simulink model "DC_Charging_Sequence_Block_testing"  (R2024b)
settings: Solver=FixedStepDiscrete  StartTime=0.0  StopTime=10.0  FixedStep=0.01  RelTol=1e-3
undefined symbols (not defined in the file or in its folder): CCM, raptor_get_safe_string, raptor_xcp_function
libraries: Raptor_lib x37
(part 1 of 2)
settings Model: RaptorUIDSize=4  Raptor_Target=CCM-58NN-112-2403  Raptor_Calloc=NonVolatile (EEPROM)  Raptor_ecuaddr=11  RaptorBuildNum=-1  Creator=noahm  LastModifiedBy=malul
settings OptimizationCC: DefaultParameterBehavior=Inlined  UseSpecifiedMinMax=on  InlineInvariantSignals=on  EnhancedBackFolding=on  PassReuseOutputArgsAs=Individual arguments  InitFltsAndDblsToZero=on  NoFixptDivByZeroProtection=on  EfficientFloat2IntCast=on  OptimizeBlockOrder=speed  DifferentSizesBufferReuse=on  OptimizationCustomize=off  EfficientTunableParamExpr=on
settings DebuggingCC: UnderspecifiedInitializationDetection=Classic  MergeDetectMultiDrivingBlocksExec=none  InheritedTsInSrcMsg=none  ParameterTunabilityLossMsg=error
settings HardwareCC: TargetIntDivRoundTo=Zero  TargetEndianess=BigEndian  ProdEqTarget=off
settings ModelReferenceCC: PropagateSignalLabelsOutOfModel=off
settings SFSimCC: MATLABDynamicMemAlloc=off
settings RTWCC: Description=Raptor (tm)  SystemTargetFile=raptor.tlc  MakeCommand=raptor_make_rtw  TemplateMakefile=raptor_tmf
settings CodeAppCC: ForceParamTrailComments=on  IgnoreCustomStorageClasses=off  MaxIdLength=100  OperatorAnnotations=on  SimulinkDataObjDesc=on  SFDataObjDesc=on  InsertBlockDesc=on
settings STFCustomTargetCC: TargetLangStandard=C99 (ISO)  MultiwordLength=256  GenerateSampleERTMain=on  CombineOutputUpdateFcns=on  CombineSignalStateStructs=on  ERTCustomFileBanners=on  SupportComplex=off  SupportContinuousTime=off  SupportNonInlinedSFcns=off  RemoveResetFunc=on  MATLABClassNameForMDSCustomization=Simulink.SoftwareTarget.ERTCustomization  SystemTargetFile=raptor.tlc
settings ERTTargetCC: TargetLangStandard=C99 (ISO)  GenerateSampleERTMain=on  ParMdlRefBuildCompliant=off  CompOptLevelCompliant=off  ConcurrentExecutionCompliant=off  CombineSignalStateStructs=on  SupportComplex=off  ModelStepFunctionPrototypeControlCompliant=off  CPPClassGenCompliant=off  UseToolchainInfoCompliant=off  ERTCustomFileTemplate=example_file_process.tlc

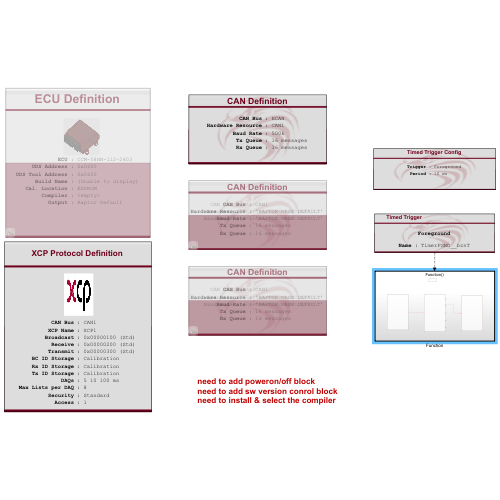
[thumbnail: Simulink's stored preview of the top-level diagram]
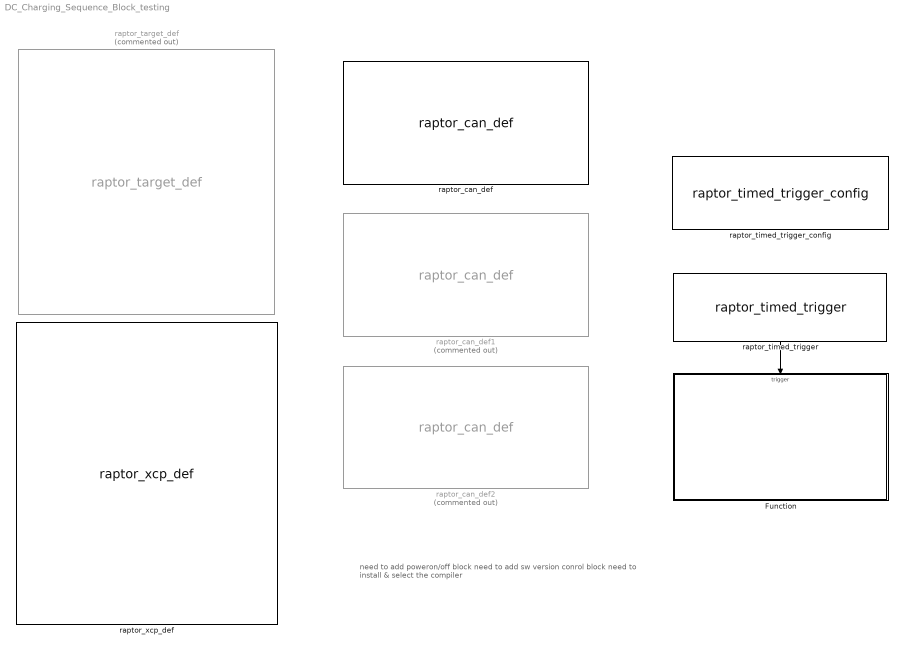
== system DC_Charging_Sequence_Block_testing ==
  note: need to add poweron/off block
      | need to add sw version conrol block
      | need to install & select the compiler
  Function : Subsystem
  raptor_can_def : Raptor_lib/CAN/raptor_can_def  canBus='HCAN'  resourceValues=CAN1|CAN2|CAN3|CAN4|CAN5|CAN6|CAN7|CAN8|(None)  resource=CAN1  baudRateValues=33k|50k|100k|125k|200k|250k|333k|500k|667k|800k|1000k  baudRate=500k  useCustomBR=0  customBR='CustomBaudRate'  enable_baud_rate_config=0  sim_func_name='ConfigureCANBaudRate'  createButton=0  updateButton=0  txQueueSize=16  rxQueueSize=16
      settings: SourceProductName=Raptor
  raptor_can_def1 : Raptor_lib/CAN/raptor_can_def  Commented=on  canBus='CAN1'  resourceValues=CAN1|CAN2|CAN3|CAN4|CAN5|CAN6|CAN7|CAN8|(None)  resource='RAPTOR MASK DEFAULT'  baudRateValues=(None)  baudRate='RAPTOR MASK DEFAULT'  useCustomBR=0  customBR='CustomBaudRate'  enable_baud_rate_config=0  sim_func_name='ConfigureCANBaudRate'  createButton=[]  updateButton=[]  txQueueSize=16  rxQueueSize=16
      settings: SourceProductName=Raptor
  raptor_can_def2 : Raptor_lib/CAN/raptor_can_def  Commented=on  canBus='CAN1'  resourceValues=CAN1|CAN2|CAN3|CAN4|CAN5|CAN6|CAN7|CAN8|(None)  resource='RAPTOR MASK DEFAULT'  baudRateValues=(None)  baudRate='RAPTOR MASK DEFAULT'  useCustomBR=0  customBR='CustomBaudRate'  enable_baud_rate_config=0  sim_func_name='ConfigureCANBaudRate'  createButton=[]  updateButton=[]  txQueueSize=16  rxQueueSize=16
      settings: SourceProductName=Raptor
  raptor_target_def : Raptor_lib/Configuration/raptor_target_def  Commented=on  targetValues=CCM-58NN-112-2403|CCM-TC377-112-2403|DISP-VC128-1901|DISP-VC320L-1402|DISP-VC320-1204|DISP-VC800-1402|DISP-VC500-1904|DISP-VC700-2003|DISP-VC300R-2004|GCM-5634M-070-1559|GCM-5634M-070-1562|EOL-58NN-176-2204|ECM-1793-196-1503|GCM-1793-196-1503|GCM-5605B-048-1906|GCM-5605B-048-2104|RCM-5743R-080-2203|RCM-5743R-080-2304|UAS-5743R-047-2102|UAS-5743R-047-2107|RCM-58NN-112-2103|RCM-58NN-112-2202|RCM-58NN-112-2208|RCM-58NN-112-2410|GCM-TC234-044-2409|GCM-TC277-106-2407|GCM-TC277-108-2406|GCM-TC337-056-2402|GCM-TC367-111-2301|HCM-5604-036-1303|HCM-5604-036-1702  target=CCM-58NN-112-2403  simpack=0  simulator=0  heap=2*1024  stack=4*1024  fgndStack=2*1024  bgndStack=2*1024  idleStack=1024  intStack=1536  sdStack=1024  appStack=1024  ecuaddr=11  uds_server_addr_ext=0  uds_server_addr=hex2dec('600')  uds_client_addr=hex2dec('650')  callocValues=Constant (FLASH)|NonVolatile (EEPROM)  calloc=NonVolatile (EEPROM)  compilerValues=[]  compiler=<empty>  setFileName=0  exeName=[raptor_get_safe_string(bdroot) '_']  addBuildNum=0  minVerChars=3  extraOutput=1  buildLocationValues=Raptor Default|Model Directory|User Defined  buildLocation=Raptor Default  exeLocation=''  exeFileButton=0  a2lLocation=''  a2lFileButton=0  rpgLocation=''  rpgFileButton=0
      settings: SourceProductName=Raptor
  raptor_timed_trigger : Raptor_lib/Triggers/raptor_timed_trigger  triggerValues=[]  trigger=Foreground  inherited=0  alwaysEnabled=1  triggerPriority=0  triggerName=FGND__bznT
      settings: SourceProductName=Raptor
  raptor_timed_trigger_config : Raptor_lib/Triggers/raptor_timed_trigger_config  triggerValues=Foreground|Background  trigger=Foreground  period=10
      settings: SourceProductName=Raptor
  raptor_xcp_def : Raptor_lib/Configuration/raptor_xcp_def  XCPname='XCP1'  canBus='CAN1'  bcID=hex2dec('100')  bcID_TypeValues=[]  bcID_Type=Standard  rxID=hex2dec('200')  rxID_TypeValues=[]  rxID_Type=Standard  txID=hex2dec('300')  txID_TypeValues=[]  txID_Type=Standard  daqRates=[5 10 100]  numODTs=8  genCANAPE=0  genVISION=0  securityValues=[]  security=Standard  dllName=raptor_XCPSecurity.dll  accessValues=[]  access=1  bcStorageValues=[]  bcStorage=Calibration  txStorageValues=[]  txStorage=Calibration  rxStorageValues=[]  rxStorage=Calibration
      settings: SourceProductName=Raptor
  wires:
  raptor_timed_trigger/1 -> Function/Trigger

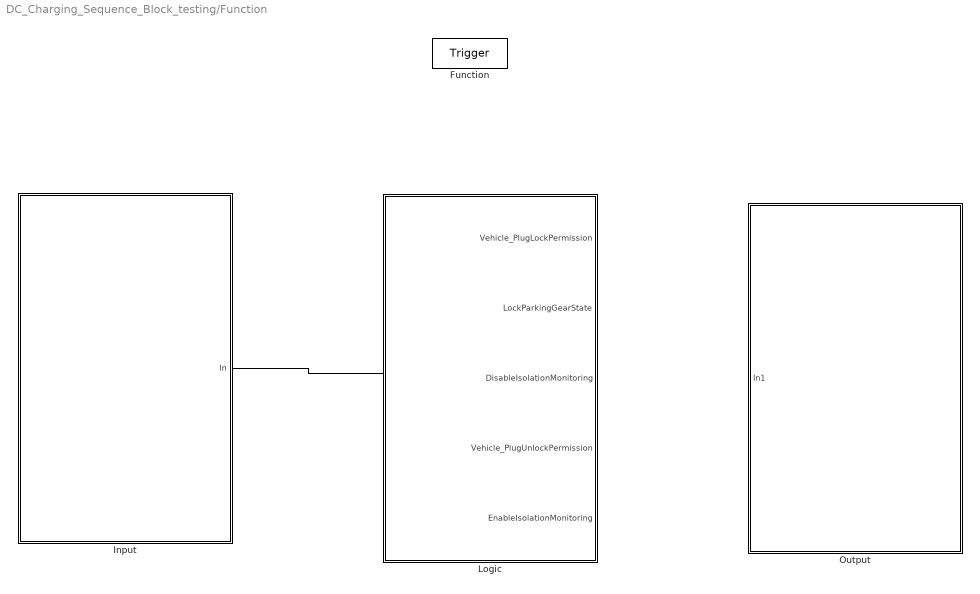
== system DC_Charging_Sequence_Block_testing/Function ==
  Function : TriggerPort  TriggerType=function-call  VariantControl=(inherit)  PortDimensions=1
  Input : Subsystem
  Logic : Subsystem
  Output : Subsystem
  wires:
  Input/1(In) -> ?
  ? -> Output/1(In1)

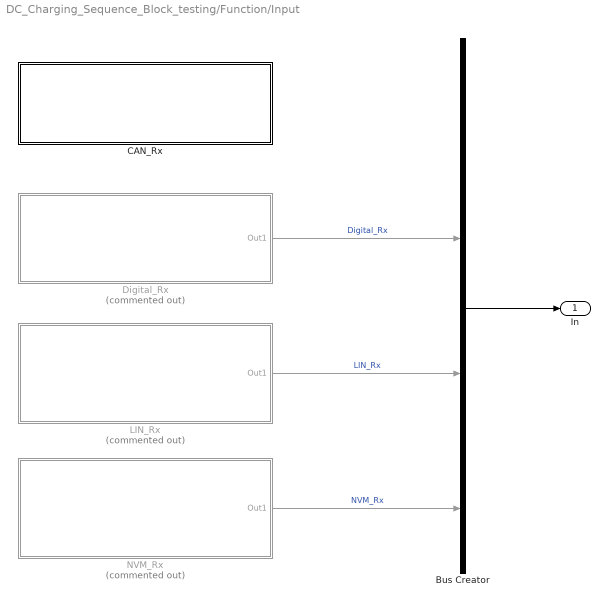
== system DC_Charging_Sequence_Block_testing/Function/Input ==
  Bus Creator : BusCreator  Inputs=4
  CAN_Rx : Subsystem
  Digital_Rx : Subsystem  Commented=on
  LIN_Rx : Subsystem  Commented=on
  NVM_Rx : Subsystem  Commented=on
  In : Outport
  wires:
  Digital_Rx/1(Out1) -> Bus Creator/2  "Digital_Rx"
  LIN_Rx/1(Out1) -> Bus Creator/3  "LIN_Rx"
  NVM_Rx/1(Out1) -> Bus Creator/4  "NVM_Rx"
  Bus Creator/1 -> In/1

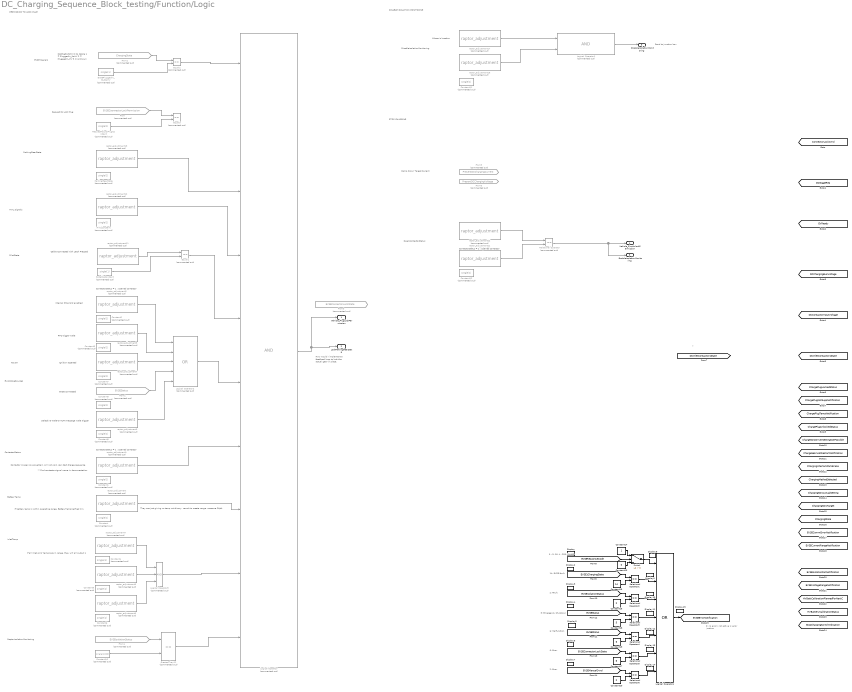
== system DC_Charging_Sequence_Block_testing/Function/Logic ==
  note: 14: EVSE fault
  note: 0 - 3: OK
      | 4 - 255: FAILED
  note: 0: no error / not active
      | 1: error / active
  note: ?
  note: DISABLE ISOLATION MONITORING
  note: PERMISSION TO LOCK PLUG
  note: Selective Wake-on-CAN message wake trigger
  note: EVSE connected
  note: Ignition asserted
  note: RTC trigger wake
  note: Internal PSU-hold enabled
  note: If all inlet pins' temps are in range, they will all output 1
  note: If battery temp is within operating range, BatteryTempVerified = 1
  note: ContactorStatus
  note: EVSE Signals
  note: ParkingGearState
  note: How would I implement a feedback loop to lock the actual gear in place.
  note: Request to Lock Plug
  note: HVIL Signals
  note: PilotState
  note: KeyOn
  note: EvccWakeSources
  note: Contactor is open so powertrain will not work, can start charge sequence
  note: ContactorStatus = 1 : opened contactor
  note: ** Find contactor signal name in documentation
  note: BatteryTemp
  note: InletTemp
  note: RaptorIsolationMonitoring
  note: ContactorStatus = 1 : opened contactor
  note: Cable Connected with Latch Pressed
  note: CcsChgPortst
      | 0 = No Cable
      | 1 = PluggedIn_NoHV
      | 2 = PluggedIn_HV
      | 3 = Unknown
  note: DisableIsolationMonitoring
  note: Ramp Down Target Current
  note: STOP CHARGING
  note: ContactorStatus = 1 : opened contactor
  note: OpenContactorStatus
  note: They are just giving us temp not binary, rework to create range. measure Dt/dt.
  note: Send to junction box
  note: Where is location
  note: 2: Fault
  note: 5: Emergency Shutdown
  note: 6: Malfunction
  note: 6: Error
  note: 2: Error
  Constant{,1..9,11..12} (12 alike) : Constant  Commented=on  Value=single(1)
  Constant10 : Constant  Commented=on  Value=single(1000)
  Constant13 : Constant  Value=0
  Constant14 : Constant  OutDataTypeStr=single
  Constant15 : Constant  Value=14
  Constant16 : Constant  Value=2
  Constant17 : Constant  Value=6
  Constant18 : Constant  Value=5
  Constant19 : Constant  Value=6
  Constant20 : Constant  Value=2
  Display{,2..15} (15 alike) : DisplayBlock  LabelPosition=Hide  Transparency=1
  EVSEPluggedIn_ButNoHV : Constant  Commented=on  Value=single(1)
  Equal1 : RelationalOperator  Commented=on  Operator===  OutDataTypeStr=boolean  RndMeth=Simplest  InputSameDT=off
  Equal2 : RelationalOperator  Commented=on  Operator===  OutDataTypeStr=boolean  RndMeth=Simplest  InputSameDT=off
  Equal3 : RelationalOperator  Commented=on  Operator===  OutDataTypeStr=boolean  RndMeth=Simplest  InputSameDT=off
  From : From  Commented=on  GotoTag=EVSECoonnectorLockPermission  TagVisibility=global
  From1 : From  Commented=on  GotoTag=EVSEStatus  TagVisibility=global
  From2 : From  Commented=on  GotoTag=ChargingState  TagVisibility=global
  From3 : From  Commented=on  GotoTag=EVSEConnectorLockState  TagVisibility=global
  From4 : From  Commented=on  GotoTag=EVSEIsolationStatus  TagVisibility=global
  From5 : From  Commented=on  GotoTag=PresentDCChargingCurrent  TagVisibility=global
  From6 : From  Commented=on  GotoTag=PresentDCChargingVoltage  TagVisibility=global
  GreaterThan11 : RelationalOperator  Commented=on  OutDataTypeStr=boolean  RndMeth=Simplest  InputSameDT=off
  HVILConstant : Constant  Commented=on  Value=single(1)
  Logical Operator : Logic  Commented=on  Inputs=10  AllPortsSameDT=off  OutDataTypeStr=boolean
  Logical Operator1 : Logic  Commented=on  AllPortsSameDT=off  OutDataTypeStr=boolean
  Logical Operator2 : Logic  Commented=on  Operator=OR  Inputs=5  AllPortsSameDT=off  OutDataTypeStr=boolean
  Logical Operator3 : Logic  Commented=on  Inputs=3  AllPortsSameDT=off  OutDataTypeStr=boolean
  Logical Operator4 : Logic  Operator=OR  Inputs=7  AllPortsSameDT=off  OutDataTypeStr=boolean
  ParkingGearState : Constant  Commented=on  Value=single(1)
  PpCableConstant : Constant  Commented=on  Value=single(1)
  Relational Operator : RelationalOperator  Commented=on  Operator===  OutDataTypeStr=boolean  RndMeth=Simplest  InputSameDT=off
  Relational Operator{1..6} (6 alike) : RelationalOperator  Operator===  OutDataTypeStr=boolean  RndMeth=Simplest  InputSameDT=off
  RequestToLockPlugConstant : Constant  Commented=on  Value=single(1)
  Switch : Switch  Criteria=u2 > Threshold  Threshold=3  SaturateOnIntegerOverflow=off  InputSameDT=off
  raptor_adjustment : Raptor_lib/Data Storage/raptor_adjustment  Commented=on  paramName='BatteryTempVerified'  nameSource=Parameter  initValue=1  dataType=single  storage=Calibration  calDispType=Number  calEnum={'False', 'True'}  calGain=1.0  calOffset=0.0  calMax=inf  calMin=-inf  calFormat='-1'  calUnit=''  calHelp=''  calAccess=1  calFunction=raptor_xcp_function(gcb)  calDispHeaders=off  calColHeaders={'Col1' 'Col2' 'Col3'}  calRowHeaders={'Row1' 'Row2' 'Row3'}
      settings: SourceProductName=Raptor
  raptor_adjustment1 : Raptor_lib/Data Storage/raptor_adjustment  Commented=on  paramName='ContactorStatus1'  nameSource=Parameter  initValue=1  dataType=single  storage=Calibration  calDispType=Number  calEnum={'False', 'True'}  calGain=1.0  calOffset=0.0  calMax=inf  calMin=-inf  calFormat='-1'  calUnit=''  calHelp=''  calAccess=1  calFunction=raptor_xcp_function(gcb)  calDispHeaders=off  calColHeaders={'Col1' 'Col2' 'Col3'}  calRowHeaders={'Row1' 'Row2' 'Row3'}
      settings: SourceProductName=Raptor
  raptor_adjustment11 : Raptor_lib/Data Storage/raptor_adjustment  Commented=on  paramName='CcsPpState_sim'  nameSource=Parameter  initValue=1  dataType=uint8  storage=Calibration  calDispType=Enumeration  calEnum={'Cable Disconnected', 'Cable Connected with Latch Pressed', 'Cable Connected with Latch Released', 'Proximity Signal is invalid'}  calGain=1.0  calOffset=0.0  calMax=inf  calMin=-inf  calFormat='-1'  calUnit=''  calHelp=''  calAccess=1  calFunction=raptor_xcp_function(gcb)  calDispHeaders=off  calColHeaders={'Col1' 'Col2' 'Col3'}  calRowHeaders={'Row1' 'Row2' 'Row3'}
      settings: SourceProductName=Raptor
  raptor_adjustment12 : Raptor_lib/Data Storage/raptor_adjustment  Commented=on  paramName='HVIL_sim'  nameSource=Parameter  initValue=1  dataType=single  storage=Calibration  calDispType=Enumeration  calEnum={'Cable Disconnected', 'Cable Connected with Latch Pressed', 'Cable Connected with Latch Released', 'Proximity Signal is invalid'}  calGain=1.0  calOffset=0.0  calMax=inf  calMin=-inf  calFormat='-1'  calUnit=''  calHelp=''  calAccess=1  calFunction=raptor_xcp_function(gcb)  calDispHeaders=off  calColHeaders={'Col1' 'Col2' 'Col3'}  calRowHeaders={'Row1' 'Row2' 'Row3'}
      settings: SourceProductName=Raptor
  raptor_adjustment13 : Raptor_lib/Data Storage/raptor_adjustment  Commented=on  paramName='ParkingGear_sim'  nameSource=Parameter  initValue=1  dataType=single  storage=Calibration  calDispType=Enumeration  calEnum={'Cable Disconnected', 'Cable Connected with Latch Pressed', 'Cable Connected with Latch Released', 'Proximity Signal is invalid'}  calGain=1.0  calOffset=0.0  calMax=inf  calMin=-inf  calFormat='-1'  calUnit=''  calHelp=''  calAccess=1  calFunction=raptor_xcp_function(gcb)  calDispHeaders=off  calColHeaders={'Col1' 'Col2' 'Col3'}  calRowHeaders={'Row1' 'Row2' 'Row3'}
      settings: SourceProductName=Raptor
  raptor_adjustment16 : Raptor_lib/Data Storage/raptor_adjustment  Commented=on  paramName='RequestDisableIsolationMonitoringConstant'  nameSource=Parameter  initValue=1  dataType=single  storage=Calibration  calDispType=Number  calEnum={'False', 'True'}  calGain=1.0  calOffset=0.0  calMax=inf  calMin=-inf  calFormat='-1'  calUnit=''  calHelp=''  calAccess=1  calFunction=raptor_xcp_function(gcb)  calDispHeaders=off  calColHeaders={'Col1' 'Col2' 'Col3'}  calRowHeaders={'Row1' 'Row2' 'Row3'}
      settings: SourceProductName=Raptor
  raptor_adjustment17 : Raptor_lib/Data Storage/raptor_adjustment  Commented=on  paramName='VehiclePlugLockConfirmation'  nameSource=Parameter  initValue=1  dataType=single  storage=Calibration  calDispType=Number  calEnum={'False', 'True'}  calGain=1.0  calOffset=0.0  calMax=inf  calMin=-inf  calFormat='-1'  calUnit=''  calHelp=''  calAccess=1  calFunction=raptor_xcp_function(gcb)  calDispHeaders=off  calColHeaders={'Col1' 'Col2' 'Col3'}  calRowHeaders={'Row1' 'Row2' 'Row3'}
      settings: SourceProductName=Raptor
  raptor_adjustment2 : Raptor_lib/Data Storage/raptor_adjustment  Commented=on  paramName='EvccWakeSources1_sim'  nameSource=Parameter  initValue=1  dataType=single  storage=Calibration  calDispType=Number  calEnum={'False', 'True'}  calGain=1.0  calOffset=0.0  calMax=inf  calMin=-inf  calFormat='-1'  calUnit=''  calHelp=''  calAccess=1  calFunction=raptor_xcp_function(gcb)  calDispHeaders=off  calColHeaders={'Col1' 'Col2' 'Col3'}  calRowHeaders={'Row1' 'Row2' 'Row3'}
      settings: SourceProductName=Raptor
  raptor_adjustment21 : Raptor_lib/Data Storage/raptor_adjustment  Commented=on  paramName='ContactorStatus1'  nameSource=Parameter  initValue=1  dataType=single  storage=Calibration  calDispType=Number  calEnum={'False', 'True'}  calGain=1.0  calOffset=0.0  calMax=inf  calMin=-inf  calFormat='-1'  calUnit=''  calHelp=''  calAccess=1  calFunction=raptor_xcp_function(gcb)  calDispHeaders=off  calColHeaders={'Col1' 'Col2' 'Col3'}  calRowHeaders={'Row1' 'Row2' 'Row3'}
      settings: SourceProductName=Raptor
  raptor_adjustment22 : Raptor_lib/Data Storage/raptor_adjustment  Commented=on  paramName='RequestToOpenContactors'  nameSource=Parameter  initValue=1  dataType=single  storage=Calibration  calDispType=Number  calEnum={'False', 'True'}  calGain=1.0  calOffset=0.0  calMax=inf  calMin=-inf  calFormat='-1'  calUnit=''  calHelp=''  calAccess=1  calFunction=raptor_xcp_function(gcb)  calDispHeaders=off  calColHeaders={'Col1' 'Col2' 'Col3'}  calRowHeaders={'Row1' 'Row2' 'Row3'}
      settings: SourceProductName=Raptor
  raptor_adjustment3 : Raptor_lib/Data Storage/raptor_adjustment  Commented=on  paramName='EvccWakeSources2_sim'  nameSource=Parameter  initValue=1  dataType=single  storage=Calibration  calDispType=Number  calEnum={'False', 'True'}  calGain=1.0  calOffset=0.0  calMax=inf  calMin=-inf  calFormat='-1'  calUnit=''  calHelp=''  calAccess=1  calFunction=raptor_xcp_function(gcb)  calDispHeaders=off  calColHeaders={'Col1' 'Col2' 'Col3'}  calRowHeaders={'Row1' 'Row2' 'Row3'}
      settings: SourceProductName=Raptor
  raptor_adjustment4 : Raptor_lib/Data Storage/raptor_adjustment  Commented=on  paramName='InletPin1TempOK'  nameSource=Parameter  initValue=1  dataType=single  storage=Calibration  calDispType=Number  calEnum={'False', 'True'}  calGain=1.0  calOffset=0.0  calMax=inf  calMin=-inf  calFormat='-1'  calUnit=''  calHelp=''  calAccess=1  calFunction=raptor_xcp_function(gcb)  calDispHeaders=off  calColHeaders={'Col1' 'Col2' 'Col3'}  calRowHeaders={'Row1' 'Row2' 'Row3'}
      settings: SourceProductName=Raptor
  raptor_adjustment5 : Raptor_lib/Data Storage/raptor_adjustment  Commented=on  paramName='InletPin2TempOK'  nameSource=Parameter  initValue=1  dataType=single  storage=Calibration  calDispType=Number  calEnum={'False', 'True'}  calGain=1.0  calOffset=0.0  calMax=inf  calMin=-inf  calFormat='-1'  calUnit=''  calHelp=''  calAccess=1  calFunction=raptor_xcp_function(gcb)  calDispHeaders=off  calColHeaders={'Col1' 'Col2' 'Col3'}  calRowHeaders={'Row1' 'Row2' 'Row3'}
      settings: SourceProductName=Raptor
  raptor_adjustment6 : Raptor_lib/Data Storage/raptor_adjustment  Commented=on  paramName='InletPin3TempOK'  nameSource=Parameter  initValue=1  dataType=single  storage=Calibration  calDispType=Number  calEnum={'False', 'True'}  calGain=1.0  calOffset=0.0  calMax=inf  calMin=-inf  calFormat='-1'  calUnit=''  calHelp=''  calAccess=1  calFunction=raptor_xcp_function(gcb)  calDispHeaders=off  calColHeaders={'Col1' 'Col2' 'Col3'}  calRowHeaders={'Row1' 'Row2' 'Row3'}
      settings: SourceProductName=Raptor
  raptor_adjustment7 : Raptor_lib/Data Storage/raptor_adjustment  Commented=on  paramName='EvccWakeSources3_sim'  nameSource=Parameter  initValue=1  dataType=single  storage=Calibration  calDispType=Number  calEnum={'False', 'True'}  calGain=1.0  calOffset=0.0  calMax=inf  calMin=-inf  calFormat='-1'  calUnit=''  calHelp=''  calAccess=1  calFunction=raptor_xcp_function(gcb)  calDispHeaders=off  calColHeaders={'Col1' 'Col2' 'Col3'}  calRowHeaders={'Row1' 'Row2' 'Row3'}
      settings: SourceProductName=Raptor
  raptor_adjustment9 : Raptor_lib/Data Storage/raptor_adjustment  Commented=on  paramName='EvccWakeSources5_sim'  nameSource=Parameter  initValue=1  dataType=single  storage=Calibration  calDispType=Number  calEnum={'False', 'True'}  calGain=1.0  calOffset=0.0  calMax=inf  calMin=-inf  calFormat='-1'  calUnit=''  calHelp=''  calAccess=1  calFunction=raptor_xcp_function(gcb)  calDispHeaders=off  calColHeaders={'Col1' 'Col2' 'Col3'}  calRowHeaders={'Row1' 'Row2' 'Row3'}
      settings: SourceProductName=Raptor
  Vehicle_PlugLockPermission : Outport
  LockParkingGearState : Outport  Port=2
  DisableIsolationMonitoring : Outport  Port=3
  Vehicle_PlugUnlockPermission : Outport  Port=4
  EnableIsolationMonitoring : Outport  Port=5
  tag scope: ChargePlugLockedStatus=global, ChargePlugNotSuppNotification=global, ChargePlugTempNotification=global, ChargePlugUnlockedStatus=global, ChargeSOCDriverSettingNotPossible=global, ChargeSessVehRestartNotification=global, ChargingInterlockParkBrake=global, ChargingMethodSelected=global, ChargingSOCActualSetting=global, ChargingSOCTarget=global, ChargingState=global, ConnectorLockCmd=global, DCChargingBusVoltage=global, DCContactorInputVoltage=global, DCInletContactor1State=global, DCStageReq=global, EVReady=global, EVSECommErrorNotification=global, EVSECurrentRangeNotification=global, EVSEErrorNotification=global, EVSEIsolationFailNotification=global, EVSEVoltageRangeNotification=global, HVBattCalibrationPlannedForNextC=global, HVBatteryCalibrationStatus=global, StopChargingSwitchIndication=global
  wires:
  Logical Operator/1 -> Vehicle_PlugLockPermission/1, LockParkingGearState/1
  Equal2/1 -> Logical Operator/1
  Logical Operator2/1 -> Logical Operator/6
  GreaterThan11/1 -> Logical Operator/10
  raptor_adjustment1/1 -> Logical Operator/7
  raptor_adjustment5/1 -> Logical Operator3/2
  raptor_adjustment4/1 -> Logical Operator3/1
  raptor_adjustment6/1 -> Logical Operator3/3
  raptor_adjustment/1 -> Logical Operator/8
  Logical Operator3/1 -> Logical Operator/9
  raptor_adjustment2/1 -> Logical Operator2/1
  raptor_adjustment3/1 -> Logical Operator2/2
  raptor_adjustment7/1 -> Logical Operator2/3
  From1/1 -> Logical Operator2/4
  raptor_adjustment9/1 -> Logical Operator2/5
  raptor_adjustment11/1 -> Equal1/1
  PpCableConstant/1 -> Equal1/2
  Equal1/1 -> Logical Operator/5
  raptor_adjustment12/1 -> Logical Operator/4
  raptor_adjustment13/1 -> Logical Operator/3
  From2/1 -> Equal2/1
  EVSEPluggedIn_ButNoHV/1 -> Equal2/2
  raptor_adjustment16/1 -> Logical Operator1/2
  Constant10/1 -> GreaterThan11/2
  raptor_adjustment17/1 -> Logical Operator1/1
  Logical Operator1/1 -> DisableIsolationMonitoring/1
  raptor_adjustment22/1 -> Relational Operator/1
  raptor_adjustment21/1 -> Relational Operator/2
  Relational Operator/1 -> Vehicle_PlugUnlockPermission/1, EnableIsolationMonitoring/1
  From/1 -> Equal3/1
  RequestToLockPlugConstant/1 -> Equal3/2
  From4/1 -> GreaterThan11/1
  Constant15/1 -> Relational Operator1/2
  Logical Operator4/1 -> [EVSEErrorNotification]
  Switch/1 -> Logical Operator4/1
  Constant16/1 -> Relational Operator2/2
  [EVSEIsolationStatus] -> Relational Operator2/1
  Relational Operator1/1 -> Logical Operator4/2
  Relational Operator2/1 -> Logical Operator4/3
  Constant18/1 -> Relational Operator3/2
  [EVSEStatus] -> Relational Operator3/1
  [EVSEStatus] -> Relational Operator4/1
  Constant19/1 -> Relational Operator4/2
  Relational Operator3/1 -> Logical Operator4/4
  Relational Operator4/1 -> Logical Operator4/5
  [EVSEConnectorLockState] -> Relational Operator5/1
  Constant17/1 -> Relational Operator5/2
  Relational Operator5/1 -> Logical Operator4/6
  Constant20/1 -> Relational Operator6/2
  [EVSEManualOvrd] -> Relational Operator6/1
  Relational Operator6/1 -> Logical Operator4/7
  [EVSEResponseCode] -> Switch/2
  [EVSE1ChargingState] -> Relational Operator1/1
  Constant14/1 -> Switch/1
  Constant13/1 -> Switch/3

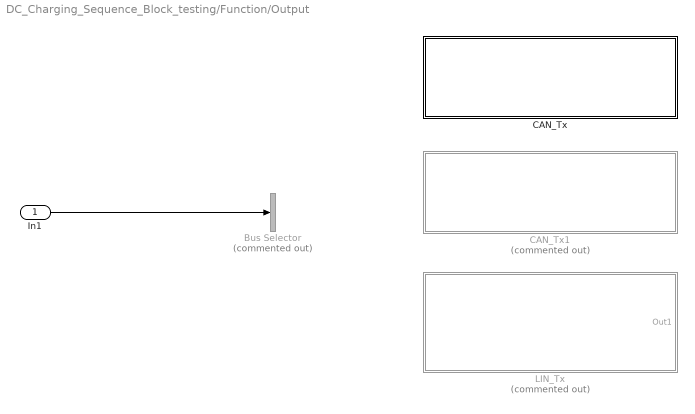
== system DC_Charging_Sequence_Block_testing/Function/Output ==
  In1 : Inport
  Bus Selector : BusSelector  Commented=on  OutputSignals=signal1,signal2
  CAN_Tx : Subsystem
  CAN_Tx1 : Subsystem  Commented=on
  LIN_Tx : Subsystem  Commented=on
  wires:
  In1/1 -> Bus Selector/1

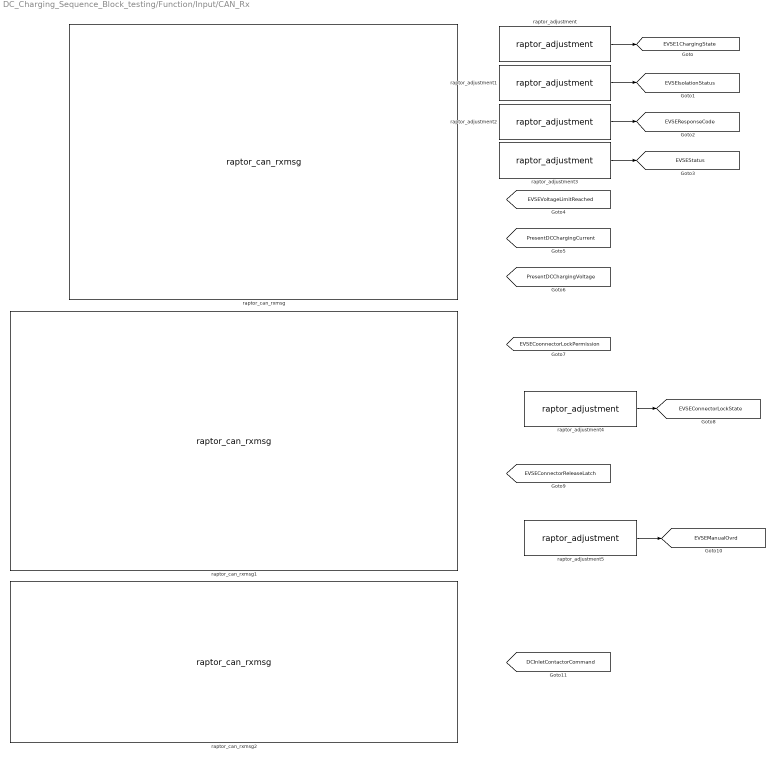
== system DC_Charging_Sequence_Block_testing/Function/Input/CAN_Rx ==
  raptor_adjustment : Raptor_lib/Data Storage/raptor_adjustment  paramName='EVSE1ChargingState'  nameSource=Parameter  initValue=13  dataType=single  storage=Calibration  calDispType=Number  calEnum={'False', 'True'}  calGain=1.0  calOffset=0.0  calMax=inf  calMin=-inf  calFormat='-1'  calUnit=''  calHelp=''  calAccess=1  calFunction=raptor_xcp_function(gcb)  calDispHeaders=off  calColHeaders={'Col1' 'Col2' 'Col3'}  calRowHeaders={'Row1' 'Row2' 'Row3'}
      settings: SourceProductName=Raptor
  raptor_adjustment1 : Raptor_lib/Data Storage/raptor_adjustment  paramName='EVSEIsoStat'  nameSource=Parameter  initValue=0  dataType=single  storage=Calibration  calDispType=Number  calEnum={'False', 'True'}  calGain=1.0  calOffset=0.0  calMax=inf  calMin=-inf  calFormat='-1'  calUnit=''  calHelp=''  calAccess=1  calFunction=raptor_xcp_function(gcb)  calDispHeaders=off  calColHeaders={'Col1' 'Col2' 'Col3'}  calRowHeaders={'Row1' 'Row2' 'Row3'}
      settings: SourceProductName=Raptor
  raptor_adjustment2 : Raptor_lib/Data Storage/raptor_adjustment  paramName='EVSEResCode'  nameSource=Parameter  initValue=3  dataType=single  storage=Calibration  calDispType=Number  calEnum={'False', 'True'}  calGain=1.0  calOffset=0.0  calMax=inf  calMin=-inf  calFormat='-1'  calUnit=''  calHelp=''  calAccess=1  calFunction=raptor_xcp_function(gcb)  calDispHeaders=off  calColHeaders={'Col1' 'Col2' 'Col3'}  calRowHeaders={'Row1' 'Row2' 'Row3'}
      settings: SourceProductName=Raptor
  raptor_adjustment3 : Raptor_lib/Data Storage/raptor_adjustment  paramName='EVSEStatus'  nameSource=Parameter  initValue=5  dataType=single  storage=Calibration  calDispType=Number  calEnum={'False', 'True'}  calGain=1.0  calOffset=0.0  calMax=inf  calMin=-inf  calFormat='-1'  calUnit=''  calHelp=''  calAccess=1  calFunction=raptor_xcp_function(gcb)  calDispHeaders=off  calColHeaders={'Col1' 'Col2' 'Col3'}  calRowHeaders={'Row1' 'Row2' 'Row3'}
      settings: SourceProductName=Raptor
  raptor_adjustment4 : Raptor_lib/Data Storage/raptor_adjustment  paramName='EVSEConLockState'  nameSource=Parameter  initValue=1  dataType=single  storage=Constant (FLASH)  calDispType=Number  calEnum={'False', 'True'}  calGain=1.0  calOffset=0.0  calMax=inf  calMin=-inf  calFormat='-1'  calUnit=''  calHelp=''  calAccess=1  calFunction=raptor_xcp_function(gcb)  calDispHeaders=off  calColHeaders={'Col1' 'Col2' 'Col3'}  calRowHeaders={'Row1' 'Row2' 'Row3'}
      settings: SourceProductName=Raptor
  raptor_adjustment5 : Raptor_lib/Data Storage/raptor_adjustment  paramName='EVSEManOvrd'  nameSource=Parameter  initValue=2  dataType=single  storage=Constant (FLASH)  calDispType=Number  calEnum={'False', 'True'}  calGain=1.0  calOffset=0.0  calMax=inf  calMin=-inf  calFormat='-1'  calUnit=''  calHelp=''  calAccess=1  calFunction=raptor_xcp_function(gcb)  calDispHeaders=off  calColHeaders={'Col1' 'Col2' 'Col3'}  calRowHeaders={'Row1' 'Row2' 'Row3'}
      settings: SourceProductName=Raptor
  raptor_can_rxmsg : Raptor_lib/CAN/raptor_can_rxmsg  canDefinition=struct('dbcFile', 'HCAN_IM40_USETHISONE.dbc','message', 'EVSE1DCS1_5F','comment', 'EVSE 1 DC Status 1','signals', {{'ChargingState','EVSECurrentLimitReached','EVSEIsolationStatus','EVSEPowerLimitReached','EVSEProcessingState','EVSEResponseCode','EVSEStatus','EVSEVoltageLimitReached','PresentDCChargingCurrent','PresentDCChargingVoltage'}},'enabled', [ 1 1 1 1 1 1 1 1 1 1;],'scaled', [ 1 1 1 1 1 1 1 1 1 1;],'canBus', '''CAN1''','messageID', [ 419084383;],'idMask', [ 536870911;],'payloadMask', [],'payloadValue', [],'period', [ 0;],'mailbox', '''''','queueSize', [ 1;],'label', [ 1;],'ver', [ 2;],'showID', [ 0;],'showRaw', [ 0;],'showRawMsg', [ 0;],'useStartVals', [ 0;],'extendedId', [ 1;],'showAge', [ 0;],'useSimFunc', [ 0;],'sim_func_name', '''''','fill', [ 0;],'editID', [ 0;],'signalOrder', [ 1;],'signalAscDes', [ 1;],'msgLength', [ 8;])  canBus='CAN1'  mailbox=''  payloadMask=[]  payloadValue=[]  idMask=hex2dec('1FFFFFFF')  queueSize=1  showID=0  label=1  fill=0  id=419084383  showRaw=0  showAge=0  signalOrder=1  signalInfo={{struct('Name', 'ChargingState','StartBit', [ 0;],'SignalSize', [ 4;],'ByteOrder', 'LittleEndian','ValueType', 'Integer','Class', 'uint8','Signed', '0','Factor', [ 1;],'Offset', [ 0;],'Min', [ 0;],'Max', [ 15;],'Units', '','Comment', 'Overall State of the DC charging system','Multiplexor', [ 0;],'Multiplexed', [ 0;],'Muxor_Name', '','MultiplexMode_Min', [],'MultiplexMode_Max', [],'StartVal', [ 0;]),struct('Name', 'EVSECurrentLimitReached','StartBit', [ 42;],'SignalSize', [ 2;],'ByteOrder', 'LittleEndian','ValueType', 'Integer','Class', 'uint8','Signed', '0','Factor', [ 1;],'Offset', [ 0;],'Min', [ 0;],'Max', [ 3;],'Units', '','Comment', 'Indicates if the output current from the EVSE has reached the negotiated current limit as determined by SPN 13160 (EVSE DC Charging Current Maximum) and SPN 13156 (Hybrid DC Charging Current Maximum).','Multiplexor', [ 0;],'Multiplexed', [ 0;],'Muxor_Name', '','MultiplexMode_Min', [],'MultiplexMode_Max', [],'StartVal', [ 0;]),struct('Name', 'EVSEIsolationStatus','StartBit', [ 4;],'SignalSize', [ 4;],'ByteOrder', 'LittleEndian','ValueType', 'Integer','Class', 'uint8','Signed', '0','Factor', [ 1;],'Offset', [ 0;],'Min', [ 0;],'Max', [ 15;],'Units', '','Comment', 'Isolation Status as returned from this instance of EVSE.','Multiplexor', [ 0;],'Multiplexed', [ 0;],'Muxor_Name', '','MultiplexMode_Min', [],'MultiplexMode_Max', [],'StartVal', [ 0;]),struct('Name', 'EVSEPowerLimitReached','StartBit', [ 44;],'SignalSize', [ 2;],'ByteOrder', 'LittleEndian','ValueType', 'Integer','Class', 'uint8','Signed', '0','Factor', [ 1;],'Offset', [ 0;],'Min', [ 0;],'Max', [ 3;],'Units', '','Comment', 'Indicates if the output power from the EVSE has reached the negotiated power limit as determined by the lower of SPN 13161 (EVSE DC Charging Power Maximum) and SPN 13157 (Hybrid DC Charging Power Maximum).','Multiplexor', [ 0;],'Multiplexed', [ 0;],'Muxor_Name', '','MultiplexMode_Min', [],'MultiplexMode_Max', [],'StartVal', [ 0;]),struct('Name', 'EVSEProcessingState','StartBit', [ 46;],'SignalSize', [ 2;],'ByteOrder', 'LittleEndian','ValueType', 'Integer','Class', 'uint8','Signed', '0','Factor', [ 1;],'Offset', [ 0;],'Min', [ 0;],'Max', [ 3;],'Units', '','Comment', 'The progress of the EVSE within its current DC Charging State, as reported by SPN 13171.','Multiplexor', [ 0;],'Multiplexed', [ 0;],'Muxor_Name', '','MultiplexMode_Min', [],'MultiplexMode_Max', [],'StartVal', [ 0;]),struct('Name', 'EVSEResponseCode','StartBit', [ 56;],'SignalSize', [ 8;],'ByteOrder', 'LittleEndian','ValueType', 'Integer','Class', 'uint8','Signed', '0','Factor', [ 1;],'Offset', [ 0;],'Min', [ 0;],'Max', [ 255;],'Units', '','Comment', 'The response code of the EVSE to the last request from the EV.','Multiplexor', [ 0;],'Multiplexed', [ 0;],'Muxor_Name', '','MultiplexMode_Min', [],'MultiplexMode_Max', [],'StartVal', [ 0;]),struct('Name', 'EVSEStatus','StartBit', [ 48;],'SignalSize', [ 4;],'ByteOrder', 'LittleEndian','ValueType', 'Integer','Class', 'uint8','Signed', '0','Factor', [ 1;],'Offset', [ 0;],'Min', [ 0;],'Max', [ 15;],'Units', '','Comment', 'Status of the DC EVSE as returned from the EVSE','Multiplexor', [ 0;],'Multiplexed', [ 0;],'Muxor_Name', '','MultiplexMode_Min', [],'MultiplexMode_Max', [],'StartVal', [ 0;]),struct('Name', 'EVSEVoltageLimitReached','StartBit', [ 40;],'SignalSize', [ 2;],'ByteOrder', 'LittleEndian','ValueType', 'Integer','Class', 'uint8','Signed', '0','Factor', [ 1;],'Offset', [ 0;],'Min', [ 0;],'Max', [ 3;],'Units', '','Comment', 'Indicates if the output voltage from the EVSE has reached the negotiated voltage limit as determined by SPN 13159 (EVSE DC Charging Voltage Maximum) and SPN 13155 (Hybrid DC Charging Voltage Maximum).','Multiplexor', [ 0;],'Multiplexed', [ 0;],'Muxor_Name', '','MultiplexMode_Min', [],'MultiplexMode_Max', [],'StartVal', [ 0;]),struct('Name', 'PresentDCChargingCurrent','StartBit', [ 24;],'SignalSize', [ 16;],'ByteOrder', 'LittleEndian','ValueType', 'Integer','Class', 'uint16','Signed', '0','Factor', [ 0.05;],'Offset', [ -1600;],'Min', [ -1600;],'Max', [ 1612.75;],'Units', 'A','Comment', 'High Voltage DC current at the output of the EVSE as measured by the EVSE','Multiplexor', [ 0;],'Multiplexed', [ 0;],'Muxor_Name', '','MultiplexMode_Min', [],'MultiplexMode_Max', [],'StartVal', [ 0;]),struct('Name', 'PresentDCChargingVoltage','StartBit', [ 8;],'SignalSize', [ 16;],'ByteOrder', 'LittleEndian','ValueType', 'Integer','Class', 'uint16','Signed', '0','Factor', [ 0.05;],'Offset', [ 0;],'Min', [ 0;],'Max', [ 3212.75;],'Units', 'V','Comment', 'High Voltage DC voltage at the output of the EVSE as measured by the EVSE','Multiplexor', [ 0;],'Multiplexed', [ 0;],'Muxor_Name', '','MultiplexMode_Min', [],'MultiplexMode_Max', [],'StartVal', [ 0;])}}  showRawMsg=0  useSimFunc=0  sim_func_name=''  useStartVals=0  extendedId=1
      settings: SourceProductName=Raptor
  raptor_can_rxmsg1 : Raptor_lib/CAN/raptor_can_rxmsg  canDefinition=struct('dbcFile', 'HCAN_IM40_USETHISONE.dbc','message', 'EVSE1S1_5F','comment', 'EVSE 1 Status 1','signals', {{'EVSEConnectorLockPermission','EVSEConnectorLockState','EVSEConnectorReleaseLatch','EVSEManualOvrd'}},'enabled', [ 1 1 1 1;],'scaled', [ 1 1 1 1;],'canBus', '''CAN1''','messageID', [ 419092063;],'idMask', [ 536870911;],'payloadMask', [],'payloadValue', [],'period', [ 0;],'mailbox', '''''','queueSize', [ 1;],'label', [ 1;],'ver', [ 2;],'showID', [ 0;],'showRaw', [ 0;],'showRawMsg', [ 0;],'useStartVals', [ 0;],'extendedId', [ 1;],'showAge', [ 0;],'useSimFunc', [ 0;],'sim_func_name', '''''','fill', [ 0;],'editID', [ 0;],'signalOrder', [ 1;],'signalAscDes', [ 1;],'msgLength', [ 8;])  canBus='CAN1'  mailbox=''  payloadMask=[]  payloadValue=[]  idMask=hex2dec('1FFFFFFF')  queueSize=1  showID=0  label=1  fill=0  id=419092063  showRaw=0  showAge=0  signalOrder=1  signalInfo={{struct('Name', 'EVSEConnectorLockPermission','StartBit', [ 8;],'SignalSize', [ 2;],'ByteOrder', 'LittleEndian','ValueType', 'Integer','Class', 'uint8','Signed', '0','Factor', [ 1;],'Offset', [ 0;],'Min', [ 0;],'Max', [ 3;],'Units', '','Comment', 'Indicates whether the connector lock is currently able to be controlled by EVSE1 Connector Lock Request, SPN 12864.','Multiplexor', [ 0;],'Multiplexed', [ 0;],'Muxor_Name', '','MultiplexMode_Min', [],'MultiplexMode_Max', [],'StartVal', [ 0;]),struct('Name', 'EVSEConnectorLockState','StartBit', [ 4;],'SignalSize', [ 3;],'ByteOrder', 'LittleEndian','ValueType', 'Integer','Class', 'uint8','Signed', '0','Factor', [ 1;],'Offset', [ 0;],'Min', [ 0;],'Max', [ 7;],'Units', '','Comment', 'Indicates the state of this EVSE Connector Lock (if present).','Multiplexor', [ 0;],'Multiplexed', [ 0;],'Muxor_Name', '','MultiplexMode_Min', [],'MultiplexMode_Max', [],'StartVal', [ 0;]),struct('Name', 'EVSEConnectorReleaseLatch','StartBit', [ 0;],'SignalSize', [ 2;],'ByteOrder', 'LittleEndian','ValueType', 'Integer','Class', 'uint8','Signed', '0','Factor', [ 1;],'Offset', [ 0;],'Min', [ 0;],'Max', [ 3;],'Units', '','Comment', 'Indicates the Release Latch status of this EVSE Connector.','Multiplexor', [ 0;],'Multiplexed', [ 0;],'Muxor_Name', '','MultiplexMode_Min', [],'MultiplexMode_Max', [],'StartVal', [ 0;]),struct('Name', 'EVSEManualOvrd','StartBit', [ 2;],'SignalSize', [ 2;],'ByteOrder', 'LittleEndian','ValueType', 'Integer','Class', 'uint8','Signed', '0','Factor', [ 1;],'Offset', [ 0;],'Min', [ 0;],'Max', [ 3;],'Units', '','Comment', 'Indicates the state of a manual override switch on the vehicle, if present. The switch may be used to disable charging and unlock the the connector.','Multiplexor', [ 0;],'Multiplexed', [ 0;],'Muxor_Name', '','MultiplexMode_Min', [],'MultiplexMode_Max', [],'StartVal', [ 0;])}}  showRawMsg=0  useSimFunc=0  sim_func_name=''  useStartVals=0  extendedId=1
      settings: SourceProductName=Raptor
  raptor_can_rxmsg2 : Raptor_lib/CAN/raptor_can_rxmsg  canDefinition=struct('dbcFile', 'HCAN_IM40_USETHISONE.dbc','message', 'EVSE1CC1_5F','comment', 'EVSE 1 Contactor Cmd 1','signals', {{'DCInletContactorCommand'}},'enabled', [ 1;],'scaled', [ 1;],'canBus', '''CAN1''','messageID', [ 419084639;],'idMask', [ 536870911;],'payloadMask', [],'payloadValue', [],'period', [ 0;],'mailbox', '''''','queueSize', [ 1;],'label', [ 1;],'ver', [ 2;],'showID', [ 0;],'showRaw', [ 0;],'showRawMsg', [ 0;],'useStartVals', [ 0;],'extendedId', [ 1;],'showAge', [ 0;],'useSimFunc', [ 0;],'sim_func_name', '''''','fill', [ 0;],'editID', [ 0;],'signalOrder', [ 1;],'signalAscDes', [ 1;],'msgLength', [ 8;])  canBus='CAN1'  mailbox=''  payloadMask=[]  payloadValue=[]  idMask=hex2dec('1FFFFFFF')  queueSize=1  showID=0  label=1  fill=0  id=419084639  showRaw=0  showAge=0  signalOrder=1  signalInfo={{struct('Name', 'DCInletContactorCommand','StartBit', [ 0;],'SignalSize', [ 2;],'ByteOrder', 'LittleEndian','ValueType', 'UNSIGNED','Class', 'uint8','Signed', [ 0;],'Factor', [ 1;],'Offset', [ 0;],'Min', [ 0;],'Max', [ 3;],'Units', '','StartVal', [ 0;],'Comment', 'Contactor command.','Multiplexed', [ 0;],'Multiplexor', [ 0;],'MultiplexMode_Min', [],'MultiplexMode_Max', [])}}  showRawMsg=0  useSimFunc=0  sim_func_name=''  useStartVals=0  extendedId=1
      settings: SourceProductName=Raptor
  tag scope: DCInletContactorCommand=global, EVSE1ChargingState=global, EVSEConnectorLockState=global, EVSEConnectorReleaseLatch=global, EVSECoonnectorLockPermission=global, EVSEIsolationStatus=global, EVSEManualOvrd=global, EVSEResponseCode=global, EVSEStatus=global, EVSEVoltageLimitReached=global, PresentDCChargingCurrent=global, PresentDCChargingVoltage=global
  wires:
  raptor_adjustment/1 -> [EVSE1ChargingState]
  raptor_adjustment1/1 -> [EVSEIsolationStatus]
  raptor_adjustment2/1 -> [EVSEResponseCode]
  raptor_adjustment3/1 -> [EVSEStatus]
  raptor_adjustment4/1 -> [EVSEConnectorLockState]
  raptor_adjustment5/1 -> [EVSEManualOvrd]

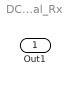
== system DC_Charging_Sequence_Block_testing/Function/Input/Digital_Rx ==
  Out1 : Outport
  wires:
  ? -> Out1/1

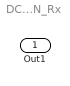
== system DC_Charging_Sequence_Block_testing/Function/Input/LIN_Rx ==
  Out1 : Outport
  wires:
  ? -> Out1/1

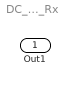
== system DC_Charging_Sequence_Block_testing/Function/Input/NVM_Rx ==
  Out1 : Outport
  wires:
  ? -> Out1/1
